simulink subsystem "subsistema_electrico_corriente_I_qs"  (R2023b)
settings: Solver=VariableStepAuto  StartTime=0.0  StopTime=10.0  RelTol=1e-3
values from neighbouring files (symbols this model uses):
  L_d = 6.6    [main.m]    (also in parametros.m = 0.0066)
  L_q = 5.8e-3    (= 0.0058)    [diagrama_polos_y_ceros_LTI.m]    (also in main.m = 5.8; parametros.m; variacion_de_parametros.m)
  lambda_m = 0.016    [main.m]    (also in parametros.m)
  P_p = 3    [diagrama_polos_y_ceros_LTI.m]    (also in main.m; parametros.m; variacion_de_parametros.m)
settings Model: Creator=nicol  LastModifiedBy=Julya

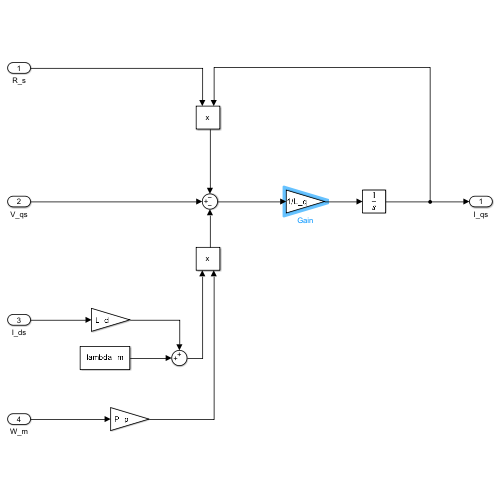
[thumbnail: Simulink's stored preview of the top-level diagram]
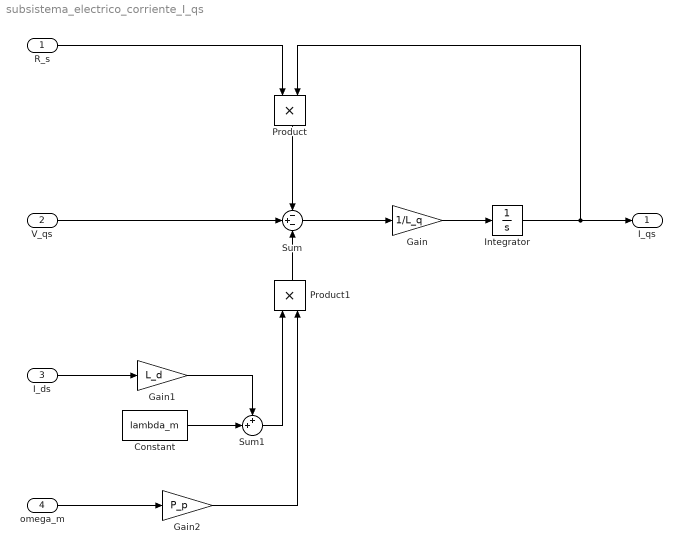
== system subsistema_electrico_corriente_I_qs ==
  R_s : Inport
  V_qs : Inport  Port=2
  I_ds : Inport  Port=3
  omega_m : Inport  Port=4
  Constant : Constant  Value=lambda_m
  Gain : Gain  Gain=1/L_q
  Gain1 : Gain  Gain=L_d
  Gain2 : Gain  Gain=P_p
  Integrator : Integrator
  Product : Product
  Product1 : Product
  Sum : Sum  Inputs=-+-
  Sum1 : Sum  Inputs=++|
  I_qs : Outport
  wires:
  I_ds/1 -> Gain1/1
  Gain1/1 -> Sum1/1
  Constant/1 -> Sum1/2
  omega_m/1 -> Gain2/1
  Gain2/1 -> Product1/2
  Sum1/1 -> Product1/1
  Product1/1 -> Sum/3
  V_qs/1 -> Sum/2
  Gain/1 -> Integrator/1
  Sum/1 -> Gain/1
  Product/1 -> Sum/1
  R_s/1 -> Product/1
  Integrator/1 -> I_qs/1, Product/2
